simulink model "thrustAllocation_2vsp_2015a"  (Simulink 8.5)
settings: Solver=ode45  SolverMode=SingleTasking  StartTime=0.0  StopTime=10.0  RelTol=1e-3
settings Model: Creator=markusfossdal  LastModifiedBy=markusfossdal  CovMetricSettings=dwe  CovHtmlReporting=off  covSaveCumulativeToWorkspaceVar=off  CovSaveSingleToWorkspaceVar=off  CovExternalEMLEnable=on
settings DataIOCC: LimitDataPoints=off  SaveFormat=Dataset  SignalLoggingSaveFormat=Dataset
settings OptimizationCC: ExpressionDepthLimit=128
settings DebuggingCC: UnderspecifiedInitializationDetection=Simplified  MergeDetectMultiDrivingBlocksExec=error  FcnCallInpInsideContextMsg=EnableAllAsError  StateNameClashWarn=none  SFUnexpectedBacktrackingDiag=error  SFNoUnconditionalDefaultTransitionDiag=error
settings HardwareCC: ProdBitPerPointer=64  ProdLargestAtomicFloat=Float  ProdIntDivRoundTo=Zero  ProdEndianess=LittleEndian  ProdHWDeviceType=Specified
settings ModelReferenceCC: PropagateSignalLabelsOutOfModel=on
settings GRTTargetCC: TargetLangStandard=C99 (ISO)  GeneratePreprocessorConditionals=Use local settings  CombineOutputUpdateFcns=on  GRTInterface=off

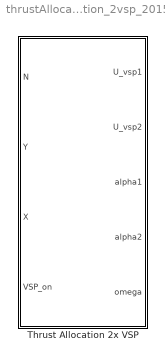
== system thrustAllocation_2vsp_2015a ==
  Thrust Allocation 2x VSP : MATLAB Function  TreatAsAtomicUnit=on
      settings: PermitHierarchicalResolution=ParametersOnly

== matlab function Thrust Allocation 2x VSP ==
  data: N input double; Y input double; X input double; U_vsp1 output double; U_vsp2 output double; alpha1 output double; alpha2 output double; omega output double; VSP_on input double
function [U_vsp1, U_vsp2, alpha1, alpha2, omega] = fcn(N,Y,X,VSP_on)

%Omega: Voith Scnheider rotational speed [rad/s]
if VSP_on
    omega = 0.3;
else
    omega = 0;
end

%Maximum forces, VS
F_max_vsp = 1.165; % [N]

%Moment arm vsp x-direction
l_vsp_x = -0.4575; %[m]

%Moment arm vsp y-direction
l_vsp_yPos = 0.0525;
l_vsp_yNeg = -0.0525;

%T-matrix thrust allocation
T = [1,0,1,0;0,1,0,1;l_vsp_yPos,l_vsp_x,l_vsp_yNeg,l_vsp_x];

%K-matrix, saturation limits for thrusters
K = [F_max_vsp 0 0 0;0 F_max_vsp 0 0; 0 0 F_max_vsp 0; 0 0 0 F_max_vsp];
TK = T*K;

%Solving the thrust allocation relation for the decomposed thrust
u = pinv(TK)*[X;Y;N];

%Assigning the decomposed thrust
U_vsp1_x = u(1,1);
U_vsp1_y = u(2,1);
U_vsp2_x = u(3,1);
U_vsp2_y = u(4,1);

%Calculating total VSP thrust
U_vsp1 = sqrt(U_vsp1_x^2 + U_vsp1_y^2);
U_vsp2 = sqrt(U_vsp2_x^2 + U_vsp2_y^2);

%Calculating thrust angle for VSP
alpha1 = atan2(U_vsp1_y,U_vsp1_x);
alpha2 = atan2(U_vsp2_y,U_vsp2_x);

    %Saturation U_vsp1
    if abs(U_vsp) > 1
        U_vsp1 = 1*sign(U_vsp1);
    end
    
    %Saturation U_vsp2
    if abs(U_vsp) > 1
        U_vsp2 = 1*sign(U_vsp2);
    end  
end %end of function
